simulink model "project"  (R2020a)
settings: Solver=VariableStepAuto  StartTime=0.0  StopTime=1000  RelTol=1e-3
values from neighbouring files (symbols this model uses):
  a = (6371+h)*1e3    (= 6871000)    [AMM_main.m]    (also in Data.m)
  A_RW = sqrt([prop1;prop2;prop3]/(prop1+prop2+prop3))    [AMM_main.m]    (also in Data.m)
  A_t = [Ax;Ay;Az;Ax;Ay;Az;A_sp;A_sp;A_sp;A_sp;]    [AMM_main.m]    (also in Data.m)
  alpha = 0.005    [AMM_main.m]    (also in Data.m = 0.5)
  cd = 2.2    [AMM_main.m]    (also in Data.m)
  horiz_ang_err = rand(3,1) - 0.5    [Data.m]
  horiz_err = 0.25*pi/180    (= 0.00436332312999)    [Data.m]
  init_DCM = DCM0_track    [AMM_main.m]    (also in Data.m = [0.097540404999410   0.957506835434298   0.970592781760616)
  init_orb = orb0_track    [AMM_main.m]    (also in Data.m = [e0,i0,O0,o0,th0])
  init_tumbl = w0_track    [AMM_main.m]    (also in Data.m = 10*pi/180*dir)
  Ir = 1e-7    (= 1e-07)    [AMM_main.m]    (also in Data.m)
  Iz = 2e-7    (= 2e-07)    [AMM_main.m]    (also in Data.m)
  J = [Jx;Jy;Jz]    [AMM_main.m]    (also in Data.m)
  K1 = .05    (= 0.05)    [AMM_main.m]    (also in Data.m)
  K2 = 0.5*K1^2    (= 0.00125)    [AMM_main.m]    (also in Data.m)
  magn_ang_err = rand(3,1) - 0.5    [Data.m]
  magn_err = 2*pi/180    (= 0.0349065850399)    [Data.m]
  max_mx = 1.19    [AMM_main.m]    (also in Data.m)
  max_my = 1.19    [AMM_main.m]    (also in Data.m)
  max_mz = 1.19    [AMM_main.m]    (also in Data.m)
  MS_freq = 1    [AMM_main.m]    (also in Data.m)
  mu = 3.986004418e14    (= 398600441800000)    [AMM_main.m]    (also in Data.m)
  n = sqrt( mu / a^3 )    [AMM_main.m]    (also in Data.m)
  rho = [rho_sMB;rho_dMB;rho_sSP;rho_dSP]    [AMM_main.m]    (also in Data.m)
  rho_air = 4.39e-16 * 1e6/1e3    (= 4.39e-13)    [AMM_main.m]    (also in Data.m)
  RW_Ir = 3.4e-4    (= 0.00034)    [AMM_main.m]    (also in Data.m)
  RW_max_momentum = 400e-3    (= 0.4)    [AMM_main.m]    (also in Data.m)
  RW_max_torque = 100e-3    (= 0.1)    [AMM_main.m]    (also in Data.m)
  wr = 100*pi/180    (= 1.74532925199)    [AMM_main.m]    (also in Data.m)
  ww_earth = 2*pi/(24*3600)*[0;0;1]    [AMM_main.m]    (also in Data.m)
libraries: vrlib x6, simulink x5, dspmtrx3 x2
(part 1 of 2)
settings Model: Creator=alejandrodemiguelmendiola  LastModifiedBy=alejandrodemiguelmendiola

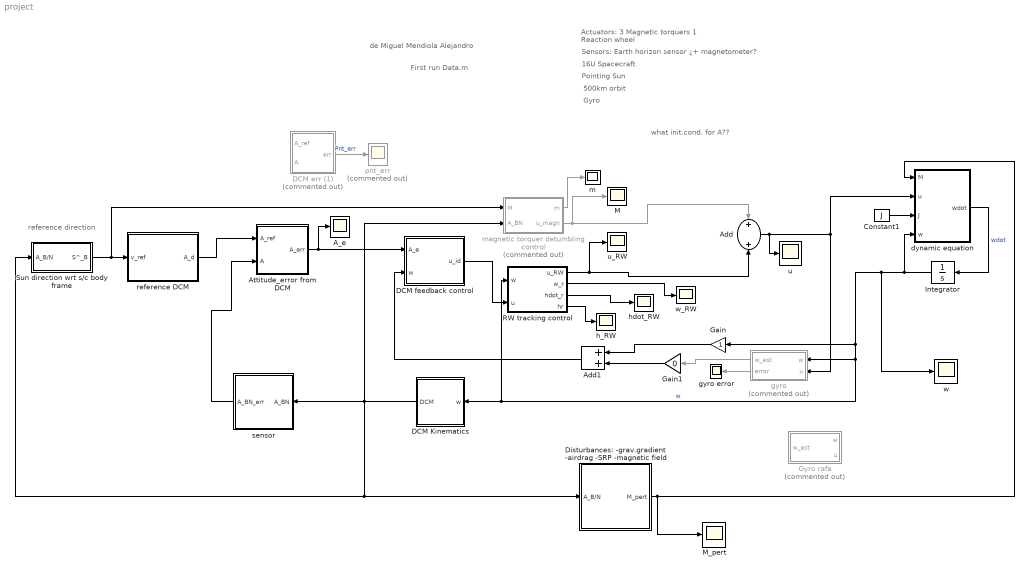
== system project ==
  note: reference direction
  note: what init.cond. for A??
  note: First run Data.m
  note: Gyro
  note: 500km orbit
  note: Pointing Sun
  note: 16U Spacecraft
  note: Sensors: Earth horizon sensor ¿+ magnetometer?
  note: Actuators: 3 Magnetic torquers
      | 		  1 Reaction wheel
  note: de Miguel Mendiola Alejandro
  A_e : Scope
  Add : Sum
  Add1 : Sum
  Attitude_error from DCM : Subsystem
  Constant1 : Constant  Value=J
  DCM Kinematics : Subsystem
  DCM err (1) : Subsystem  Commented=on
  DCM feedback control : Subsystem
  Disturbances: -grav.gradient -airdrag -SRP -magnetic field : Subsystem
  Gain : Gain
  Gain1 : Gain  Gain=0
  Gyro rafa : Subsystem  Commented=on
  Integrator : Integrator  InitialCondition=[1;1;1]*1e-3
  M : Scope
  M_pert : Scope
  RW tracking control : Subsystem
  Sun direction wrt s/c body frame : Subsystem
  dynamic equation : MATLAB Function  TreatAsAtomicUnit=on
  gyro : Subsystem  Commented=on
  gyro error : Scope
  h_RW : Scope
  hdot_RW : Scope
  m : Scope
  magnetic torquer detumbling control : Subsystem  Commented=on
  pnt_err : Scope  Commented=on
  reference DCM : Subsystem
  sensor : Subsystem
  u : Scope
  u_RW : Scope
  w : Scope
  w_RW : Scope
  wires:
  dynamic equation/1(wdot) -> Integrator/1  "wdot"
  Integrator/1 -> RW tracking control/1(w), DCM Kinematics/1(w), gyro/1(w), Gain/1, w/1, dynamic equation/4(w)  "w"
  Disturbances: -grav.gradient -airdrag -SRP -magnetic field/1(M_pert) -> dynamic equation/1(M), M_pert/1
  magnetic torquer detumbling control/2(u_magn) -> M/1, Add/1
  RW tracking control/1(u_RW) -> Add/2, u_RW/1
  Add/1 -> u/1, gyro/2(u), dynamic equation/2(u)
  gyro/2(error) -> gyro error/1
  RW tracking control/2(w_r) -> w_RW/1
  RW tracking control/3(hdot_r) -> hdot_RW/1
  Constant1/1 -> dynamic equation/3(J)
  RW tracking control/4(hr) -> h_RW/1
  Add1/1 -> DCM feedback control/2(w)
  Gain1/1 -> Add1/2
  gyro/1(w_est) -> Gain1/1
  Gain/1 -> Add1/1
  magnetic torquer detumbling control/1(m) -> m/1
  Sun direction wrt s/c body frame/1(S^_B) -> magnetic torquer detumbling control/1(M), reference DCM/1(v_ref)
  reference DCM/1(A_d) -> Attitude_error from DCM/1(A_ref)
  DCM feedback control/1(u_id) -> RW tracking control/2(u)
  DCM Kinematics/1(DCM) -> Sun direction wrt s/c body frame/1(A_B/N), Disturbances: -grav.gradient -airdrag -SRP -magnetic field/1(A_B/N), sensor/1(A_BN), magnetic torquer detumbling control/2(A_BN)
  Attitude_error from DCM/1(A_err) -> A_e/1, DCM feedback control/1(A_e)
  DCM err (1)/1(err) -> pnt_err/1  "Pnt_err"
  sensor/1(A_BN_err) -> Attitude_error from DCM/2(A)

== system project/Attitude_error from DCM ==
  A_ref : Inport
  A : Inport  Port=2
  Identity Matrix : dspmtrx3/Identity Matrix  Inherit=off  N=3  Ts=1  dataType=double  isSigned=on  wordLen=16  udDataType=sfix(16)  fracBitsMode=Best precision  numFracBits=15  OutDataTypeStr=double  LastOutDataTypeStr=double
  Matrix Multiply1 : Product  Multiplication=Matrix(*)
  Sum : Sum  Inputs=-+|
  Transpose1 : Math  Operator=transpose  SaturateOnIntegerOverflow=on
  A_err : Outport
  wires:
  Identity Matrix/1 -> Sum/1
  Matrix Multiply1/1 -> Sum/2
  A_ref/1 -> Transpose1/1
  Transpose1/1 -> Matrix Multiply1/2
  A/1 -> Matrix Multiply1/1
  Sum/1 -> A_err/1

== system project/DCM Kinematics ==
  w : Inport
  Integrator : Integrator  InitialCondition=init_DCM
  Iterative Orthonormalization : Subsystem
  Product1 : Product  Multiplication=Matrix(*)
  Unary Minus : UnaryMinus
  hat : MATLAB Function  TreatAsAtomicUnit=on
  DCM : Outport
  wires:
  Unary Minus/1 -> Integrator/1  "Adot"
  hat/1(w_hat) -> Product1/1
  Product1/1 -> Unary Minus/1
  w/1 -> hat/1(w)
  Iterative Orthonormalization/1(A_Ortho) -> Product1/2, DCM/1  "A_ortho"
  Integrator/1 -> Iterative Orthonormalization/1(A)  "A"

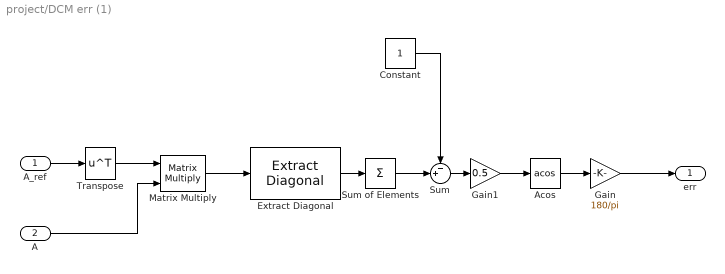
== system project/DCM err (1) ==
  A_ref : Inport
  A : Inport  Port=2
  Acos : Trigonometry  Operator=acos
  Constant : Constant
  Extract Diagonal : dspmtrx3/Extract Diagonal
      settings: SourceProductBaseCode=DS
  Gain : Gain  Gain=180/pi
  Gain1 : Gain  Gain=0.5
  Matrix Multiply : Product  Multiplication=Matrix(*)
  Sum : Sum  Inputs=-+|
  Sum of Elements : Sum  Inputs=+
  Transpose : Math  Operator=transpose  SaturateOnIntegerOverflow=on
  err : Outport
  wires:
  Transpose/1 -> Matrix Multiply/1
  Matrix Multiply/1 -> Extract Diagonal/1
  Extract Diagonal/1 -> Sum of Elements/1
  A/1 -> Matrix Multiply/2
  A_ref/1 -> Transpose/1
  Sum/1 -> Gain1/1
  Acos/1 -> Gain/1
  Sum of Elements/1 -> Sum/2
  Constant/1 -> Sum/1
  Gain/1 -> err/1
  Gain1/1 -> Acos/1

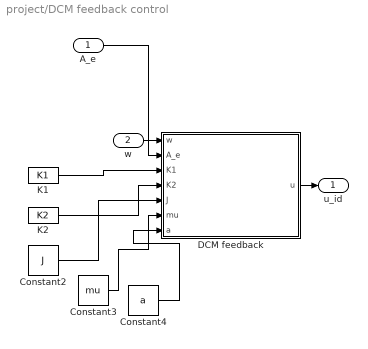
== system project/DCM feedback control ==
  A_e : Inport
  w : Inport  Port=2
  Constant2 : Constant  Value=J
  Constant3 : Constant  Value=mu
  Constant4 : Constant  Value=a
  DCM feedback : MATLAB Function  TreatAsAtomicUnit=on
  K1 : Constant  Value=K1
  K2 : Constant  Value=K2
  u_id : Outport
  wires:
  DCM feedback/1(u) -> u_id/1
  A_e/1 -> DCM feedback/2(A_e)
  Constant3/1 -> DCM feedback/6(mu)
  Constant2/1 -> DCM feedback/5(J)
  Constant4/1 -> DCM feedback/7(a)
  K2/1 -> DCM feedback/4(K2)
  w/1 -> DCM feedback/1(w)
  K1/1 -> DCM feedback/3(K1)

== system project/Disturbances: -grav.gradient -airdrag -SRP -magnetic field ==
  A_B/N : Inport
  Add : Sum  Inputs=++++
  SRP moment : Subsystem
  air drag : Subsystem
  gravity gradient : Subsystem
  magnetic torque : Subsystem
  M_pert : Outport
  wires:
  magnetic torque/1(magnetic torque M) -> Add/1
  SRP moment/1(T_srp) -> Add/2
  gravity gradient/1(G) -> Add/4
  Add/1 -> M_pert/1
  air drag/1(M_drag) -> Add/3
  A_B/N/1 -> magnetic torque/1(A_BN), SRP moment/1(A_B/N), gravity gradient/1(A_BN), air drag/1(A_B/N)

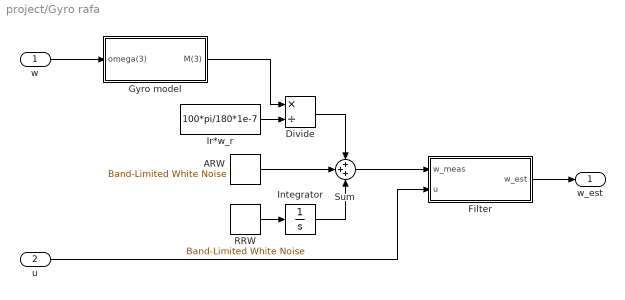
== system project/Gyro rafa ==
  w : Inport
  u : Inport  Port=2
  ARW : simulink/Sources/Band-Limited White Noise  Cov=1.9039e-09  Ts=0.0038168  seed=[23341]
  Divide : Product  Inputs=*/
  Filter : Subsystem
  Gyro model : Subsystem
  Integrator : Integrator  InitialCondition=pi/180/3600*[1 1 1]'
  Ir*w_r : Constant  Value=100*pi/180*1e-7
  RRW : simulink/Sources/Band-Limited White Noise  Cov=5.5423e-10  Ts=0.0038168  seed=[23341]
  Sum : Sum  Inputs=+++
  w_est : Outport
  wires:
  w/1 -> Gyro model/1(omega(3))
  Divide/1 -> Sum/1
  Sum/1 -> Filter/1(w_meas)
  Ir*w_r/1 -> Divide/2
  Gyro model/1(M(3)) -> Divide/1
  u/1 -> Filter/2(u)
  Filter/1(w_est) -> w_est/1
  ARW/1 -> Sum/2
  RRW/1 -> Integrator/1
  Integrator/1 -> Sum/3

== system project/RW tracking control ==
  w : Inport
  u : Inport  Port=2
  detumblingl control of 1 RW : Subsystem
  u_RW : Outport
  w_r : Outport  Port=2
  hdot_r : Outport  Port=3
  hr : Outport  Port=4
  wires:
  w/1 -> detumblingl control of 1 RW/1(w)
  detumblingl control of 1 RW/2(w_r) -> w_r/1
  detumblingl control of 1 RW/1(u_c) -> u_RW/1
  detumblingl control of 1 RW/4(hr) -> hr/1
  detumblingl control of 1 RW/3(hdot_r) -> hdot_r/1
  u/1 -> detumblingl control of 1 RW/2(u)

== system project/Sun direction wrt s//c body frame ==
  A_B/N : Inport
  Clock : Clock
  Product3 : Product  Multiplication=Matrix(*)
  Sun's direction : MATLAB Function  TreatAsAtomicUnit=on
  S^_B : Outport
  wires:
  Product3/1 -> S^_B/1
  A_B/N/1 -> Product3/1
  Clock/1 -> Sun's direction/1(t)
  Sun's direction/1(S_N) -> Product3/2  "S^_N"

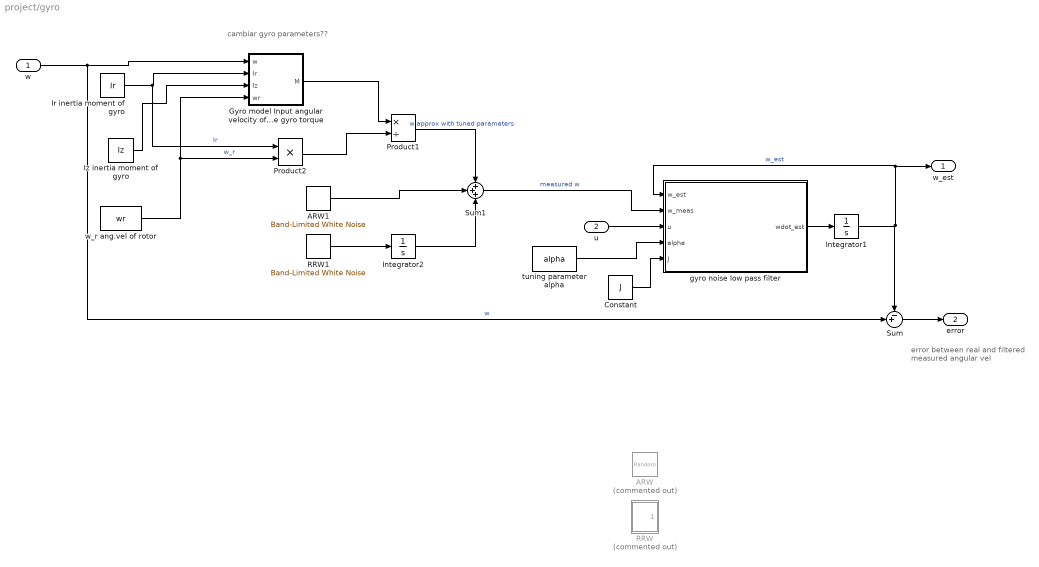
== system project/gyro ==
  note: cambiar gyro parameters??
  note: error between real
      | and filtered measured angular vel
  w : Inport
  u : Inport  Port=2
  ARW : RandomNumber  Commented=on  Variance=[1;1;1]*0.0025*pi/180  SampleTime=1/900  VectorParams1D=off
  ARW1 : simulink/Sources/Band-Limited White Noise  Cov=1.9039e-09  Ts=0.0038168  seed=[23341]
  Constant : Constant  Value=J
  Gyro model Input angular velocity of the spacecraft with output the gyro torque : Subsystem
  Integrator1 : Integrator  InitialCondition=init_tumbl
  Integrator2 : Integrator  InitialCondition=pi/180/3600*[1,1,1]'
  Ir inertia moment of gyro : Constant  Value=Ir
  Iz inertia moment of gyro : Constant  Value=Iz
  Product1 : Product  Inputs=*/
  Product2 : Product  Inputs=**
  RRW : Subsystem  Commented=on
  RRW1 : simulink/Sources/Band-Limited White Noise  Cov=5.5423e-10  Ts=0.0038168  seed=[23341]
  Sum : Sum  Inputs=-+|
  Sum1 : Sum  Inputs=+++
  gyro noise low pass filter : MATLAB Function  TreatAsAtomicUnit=on
  tuning parameter alpha : Constant  Value=alpha
  w_r ang.vel of rotor : Constant  Value=wr
  w_est : Outport
  error : Outport  Port=2
  wires:
  gyro noise low pass filter/1(wdot_est) -> Integrator1/1
  u/1 -> gyro noise low pass filter/3(u)
  tuning parameter alpha/1 -> gyro noise low pass filter/4(alpha)
  Sum/1 -> error/1
  Product2/1 -> Product1/2
  w/1 -> Gyro model Input angular velocity of the spacecraft with output the gyro torque/1(w), Sum/2  "w"
  Product1/1 -> Sum1/1  "w approx with tuned parameters"
  Integrator1/1 -> Sum/1, w_est/1, gyro noise low pass filter/1(w_est)  "w_est"
  Ir inertia moment of gyro/1 -> Product2/1, Gyro model Input angular velocity of the spacecraft with output the gyro torque/2(Ir)  "Ir"
  w_r ang.vel of rotor/1 -> Product2/2, Gyro model Input angular velocity of the spacecraft with output the gyro torque/4(wr)  "w_r"
  Iz inertia moment of gyro/1 -> Gyro model Input angular velocity of the spacecraft with output the gyro torque/3(Iz)
  Sum1/1 -> gyro noise low pass filter/2(w_meas)  "measured w"
  Gyro model Input angular velocity of the spacecraft with output the gyro torque/1(M) -> Product1/1
  Constant/1 -> gyro noise low pass filter/5(J)
  ARW1/1 -> Sum1/2
  RRW1/1 -> Integrator2/1
  Integrator2/1 -> Sum1/3

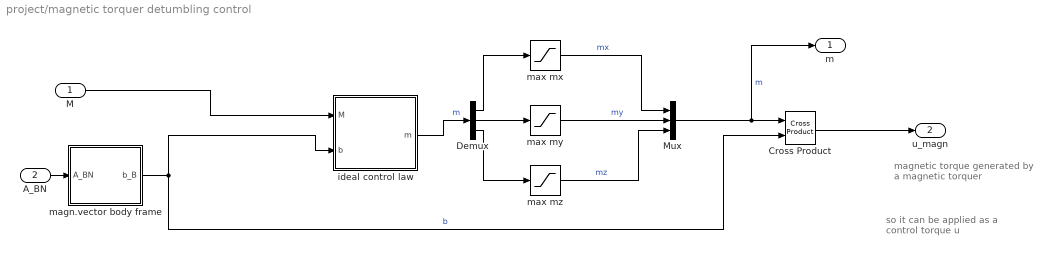
== system project/magnetic torquer detumbling control ==
  note: so it can be applied
      | as a control torque u
  note: magnetic torque
      | generated by a
      | magnetic torquer
  M : Inport
  A_BN : Inport  Port=2
  Cross Product : vrlib/Utilities/Cross Product
  Demux : Demux  Outputs=3
  Mux : Mux  Inputs=3
  ideal control law : MATLAB Function  TreatAsAtomicUnit=on
  magn.vector body frame : Subsystem
  max mx : Saturate  UpperLimit=max_mx  LowerLimit=-max_mx  ZeroCross=off
  max my : Saturate  UpperLimit=max_my  LowerLimit=-max_my  ZeroCross=off
  max mz : Saturate  UpperLimit=max_mz  LowerLimit=-max_mz  ZeroCross=off
  m : Outport
  u_magn : Outport  Port=2
  wires:
  ideal control law/1(m) -> Demux/1  "m"
  magn.vector body frame/1(b_B) -> ideal control law/2(b), Cross Product/2  "b"
  Mux/1 -> m/1, Cross Product/1  "m"
  Cross Product/1 -> u_magn/1
  max mx/1 -> Mux/1  "mx"
  max my/1 -> Mux/2  "my"
  max mz/1 -> Mux/3  "mz"
  Demux/1 -> max mx/1
  Demux/2 -> max my/1
  Demux/3 -> max mz/1
  M/1 -> ideal control law/1(M)
  A_BN/1 -> magn.vector body frame/1(A_BN)

== system project/reference DCM ==
  v_ref : Inport
  Constant2 : Constant  Value=a
  DCM_ref : MATLAB Function  TreatAsAtomicUnit=on
  Terminator : Terminator
  s/c position for a given orbit : Subsystem
  A_d : Outport
  wires:
  DCM_ref/1(A_BN) -> A_d/1
  Constant2/1 -> s/c position for a given orbit/1(a)
  v_ref/1 -> DCM_ref/1(v_ref)
  s/c position for a given orbit/1(r_N) -> DCM_ref/2(r_sc)
  s/c position for a given orbit/2(v_N) -> Terminator/1  "v_inertial"

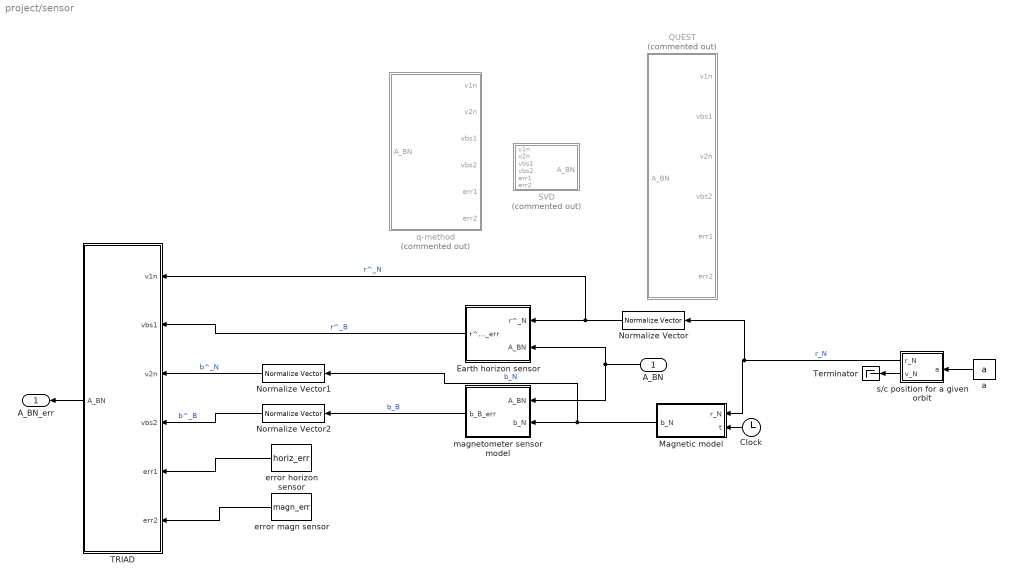
== system project/sensor ==
  A_BN : Inport
  Clock : Clock
  Earth horizon sensor : Subsystem
  Magnetic model : MATLAB Function  TreatAsAtomicUnit=on
  Normalize Vector : vrlib/Utilities/Normalize Vector  maxzero=0
  Normalize Vector1 : vrlib/Utilities/Normalize Vector  maxzero=0
  Normalize Vector2 : vrlib/Utilities/Normalize Vector  maxzero=0
  QUEST : MATLAB Function  Commented=on  TreatAsAtomicUnit=on
  SVD : MATLAB Function  Commented=on  TreatAsAtomicUnit=on
  TRIAD : MATLAB Function  TreatAsAtomicUnit=on
  Terminator : Terminator
  a : Constant  Value=a
  error horizon sensor : Constant  Value=horiz_err
  error magn sensor : Constant  Value=magn_err
  magnetometer sensor model : Subsystem
  q-method : MATLAB Function  Commented=on  TreatAsAtomicUnit=on
  s/c position for a given orbit : Subsystem
  A_BN_err : Outport
  wires:
  A_BN/1 -> Earth horizon sensor/2(A_BN), magnetometer sensor model/1(A_BN)
  Magnetic model/1(b_N) -> Normalize Vector1/1, magnetometer sensor model/2(b_N)  "b_N"
  Clock/1 -> Magnetic model/2(t)
  magnetometer sensor model/1(b_B_err) -> Normalize Vector2/1  "b_B"
  Earth horizon sensor/1(r^_B_err) -> TRIAD/2(vbs1)  "r^_B"
  TRIAD/1(A_BN) -> A_BN_err/1
  s/c position for a given orbit/2(v_N) -> Terminator/1
  a/1 -> s/c position for a given orbit/1(a)
  s/c position for a given orbit/1(r_N) -> Normalize Vector/1, Magnetic model/1(r_N)  "r_N"
  Normalize Vector/1 -> TRIAD/1(v1n), Earth horizon sensor/1(r^_N)  "r^_N"
  Normalize Vector2/1 -> TRIAD/4(vbs2)  "b^_B"
  Normalize Vector1/1 -> TRIAD/3(v2n)  "b^_N"
  error horizon sensor/1 -> TRIAD/5(err1)
  error magn sensor/1 -> TRIAD/6(err2)

== system project/DCM Kinematics/Iterative Orthonormalization ==
  note: Uncomment if needed
      | With 2 blocks working:
      | Error ~1e-16 up to t=1e6
      | Error ~1e-14 up to t=1e7
  A : Inport
  Ortho DCM : Subsystem
  Ortho DCM1 : Subsystem
  Ortho DCM2 : Subsystem  Commented=through
  Ortho DCM3 : Subsystem  Commented=through
  Ortho DCM4 : Subsystem  Commented=through
  A_Ortho : Outport
  wires:
  Ortho DCM1/1(A_ortho) -> Ortho DCM2/1(A)
  Ortho DCM/1(A_ortho) -> Ortho DCM1/1(A)
  Ortho DCM3/1(A_ortho) -> Ortho DCM4/1(A)
  Ortho DCM2/1(A_ortho) -> Ortho DCM3/1(A)
  A/1 -> Ortho DCM/1(A)
  Ortho DCM4/1(A_ortho) -> A_Ortho/1

== system project/Disturbances: -grav.gradient -airdrag -SRP -magnetic field/SRP moment ==
  A_B/N : Inport
  Area : Constant  Value=A_t
  SRP disturbance torque : MATLAB Function  TreatAsAtomicUnit=on
  Sun direction wrt s/c body frame : Subsystem
  optical properties : Constant  Value=rho
  T_srp : Outport
  wires:
  A_B/N/1 -> Sun direction wrt s/c body frame/1(A_B/N)
  SRP disturbance torque/1(T_srp) -> T_srp/1
  Sun direction wrt s/c body frame/1(S^_B) -> SRP disturbance torque/1(S_B)
  Area/1 -> SRP disturbance torque/2(A)
  optical properties/1 -> SRP disturbance torque/3(rho)

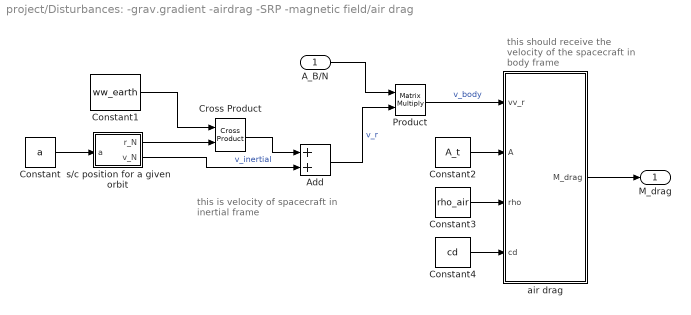
== system project/Disturbances: -grav.gradient -airdrag -SRP -magnetic field/air drag ==
  note: this is velocity
      | of spacecraft in
      | inertial frame
  note: this should receive the
      | velocity of the spacecraft
      | in body frame
  A_B/N : Inport
  Add : Sum
  Constant : Constant  Value=a
  Constant1 : Constant  Value=ww_earth
  Constant2 : Constant  Value=A_t
  Constant3 : Constant  Value=rho_air
  Constant4 : Constant  Value=cd
  Cross Product : vrlib/Utilities/Cross Product
  Product : Product  Multiplication=Matrix(*)
  air drag : MATLAB Function  TreatAsAtomicUnit=on
  s/c position for a given orbit : Subsystem
  M_drag : Outport
  wires:
  air drag/1(M_drag) -> M_drag/1
  A_B/N/1 -> Product/1
  Product/1 -> air drag/1(vv_r)  "v_body"
  Constant/1 -> s/c position for a given orbit/1(a)
  s/c position for a given orbit/1(r_N) -> Cross Product/2
  Constant1/1 -> Cross Product/1
  Cross Product/1 -> Add/1
  s/c position for a given orbit/2(v_N) -> Add/2  "v_inertial"
  Add/1 -> Product/2  "v_r"
  Constant2/1 -> air drag/2(A)
  Constant4/1 -> air drag/4(cd)
  Constant3/1 -> air drag/3(rho)

== system project/Disturbances: -grav.gradient -airdrag -SRP -magnetic field/gravity gradient ==
  A_BN : Inport
  A_N/L : Subsystem
  Product : Product  Multiplication=Matrix(*)
  gravity gradient : MATLAB Function  TreatAsAtomicUnit=on
  mean motion : Constant  Value=n
  moment of inertia : Constant  Value=J
  G : Outport
  wires:
  gravity gradient/1(G) -> G/1
  A_N/L/1(A_N/L) -> Product/2
  A_BN/1 -> Product/1
  Product/1 -> gravity gradient/1(A_BL)
  moment of inertia/1 -> gravity gradient/2(J)
  mean motion/1 -> gravity gradient/3(n)

== system project/Disturbances: -grav.gradient -airdrag -SRP -magnetic field/magnetic torque ==
  A_BN : Inport
  Cross Product : vrlib/Utilities/Cross Product
  m (worst case scenario) : Constant  Value=[0.1;0.1;0.1]
  m (from labs) : Constant  Commented=on  Value=[0.01;0.05;0.01]
  magnetic model : Subsystem
  magnetic torque M : Outport
  wires:
  magnetic model/1(b_B) -> Cross Product/2  "b_B"
  m (worst case scenario)/1 -> Cross Product/1
  Cross Product/1 -> magnetic torque M/1  "M"
  A_BN/1 -> magnetic model/1(A_BN)

== system project/Gyro rafa/Filter ==
  w_meas : Inport
  u : Inport  Port=2
  Integrator : Integrator  InitialCondition=[-0.0157; -0.1329; 0.1121]
  MATLAB Function : MATLAB Function  TreatAsAtomicUnit=on
  w_est : Outport
  wires:
  MATLAB Function/1(west_dot) -> Integrator/1
  Integrator/1 -> w_est/1, MATLAB Function/3(w_est)
  w_meas/1 -> MATLAB Function/1(w_meas)
  u/1 -> MATLAB Function/2(u)

== system project/Gyro rafa/Gyro model ==
  omega(3) : Inport
  Integrator : Integrator  InitialCondition=zeros(6,1)
  MATLAB Function : MATLAB Function  TreatAsAtomicUnit=on
  Scope : Scope
  Scope1 : Scope
  M(3) : Outport
  wires:
  MATLAB Function/2(M) -> M(3)/1
  omega(3)/1 -> MATLAB Function/2(w)
  MATLAB Function/1(x_dot) -> Scope/1, Integrator/1
  Integrator/1 -> Scope1/1, MATLAB Function/1(x)

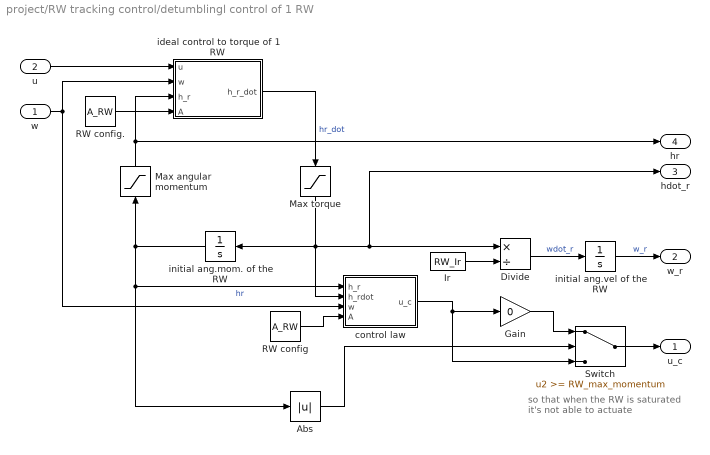
== system project/RW tracking control/detumblingl control of 1 RW ==
  note: so that when the RW is saturated
      | it's not able to actuate
  w : Inport
  u : Inport  Port=2
  Abs : Abs
  Divide : Product  Inputs=*/
  Gain : Gain  Gain=0
  Ir : Constant  Value=RW_Ir
  Max angular momentum : Saturate  UpperLimit=RW_max_momentum  LowerLimit=-RW_max_momentum
  Max torque : Saturate  UpperLimit=RW_max_torque  LowerLimit=-RW_max_torque  ZeroCross=off
  RW config : Constant  Value=A_RW
  RW config. : Constant  Value=A_RW
  Switch : Switch  Threshold=RW_max_momentum
  control law : MATLAB Function  TreatAsAtomicUnit=on
  ideal control to torque of 1 RW : MATLAB Function  TreatAsAtomicUnit=on
  "initial ang.mom. of the RW " : Integrator
  initial ang.vel of the RW : Integrator
  u_c : Outport
  w_r : Outport  Port=2
  hdot_r : Outport  Port=3
  hr : Outport  Port=4
  wires:
  u/1 -> ideal control to torque of 1 RW/1(u)
  w/1 -> ideal control to torque of 1 RW/2(w), control law/3(w)
  ideal control to torque of 1 RW/1(h_r_dot) -> Max torque/1  "hr_dot"
  "initial ang.mom. of the RW "/1 -> Max angular momentum/1, Abs/1, control law/1(h_r)  "hr"
  Max torque/1 -> "initial ang.mom. of the RW "/1, control law/2(h_rdot), hdot_r/1, Divide/1
  Max angular momentum/1 -> hr/1, ideal control to torque of 1 RW/3(h_r)
  Ir/1 -> Divide/2
  Divide/1 -> initial ang.vel of the RW/1  "wdot_r"
  initial ang.vel of the RW/1 -> w_r/1  "w_r"
  RW config/1 -> control law/4(A)
  RW config./1 -> ideal control to torque of 1 RW/4(A)
  Abs/1 -> Switch/2
  Switch/1 -> u_c/1
  control law/1(u_c) -> Gain/1, Switch/3
  Gain/1 -> Switch/1

== system project/gyro/Gyro model Input angular velocity of the spacecraft with output the gyro torque ==
  w : Inport
  Ir : Inport  Port=2
  Iz : Inport  Port=3
  wr : Inport  Port=4
  Integrator2 : Integrator  InitialCondition=[0;0;0;0;0;0]
  MATLAB Function1 : MATLAB Function  TreatAsAtomicUnit=on
  M : Outport
  wires:
  Integrator2/1 -> MATLAB Function1/4(x)
  MATLAB Function1/1(x_dot) -> Integrator2/1
  w/1 -> MATLAB Function1/5(w)
  MATLAB Function1/2(M) -> M/1
  Ir/1 -> MATLAB Function1/1(Ir)
  Iz/1 -> MATLAB Function1/2(Iz)
  wr/1 -> MATLAB Function1/3(w_r)

== system project/gyro/RRW ==
  Integrator2 : Integrator  InitialCondition=pi/180/3600*[1;1;1]
  Random Number : RandomNumber  Variance=1.5e-8*[1;1;1]  SampleTime=1/900  VectorParams1D=off
  RRW : Outport
  wires:
  Integrator2/1 -> RRW/1  "b"
  Random Number/1 -> Integrator2/1  "bdot"

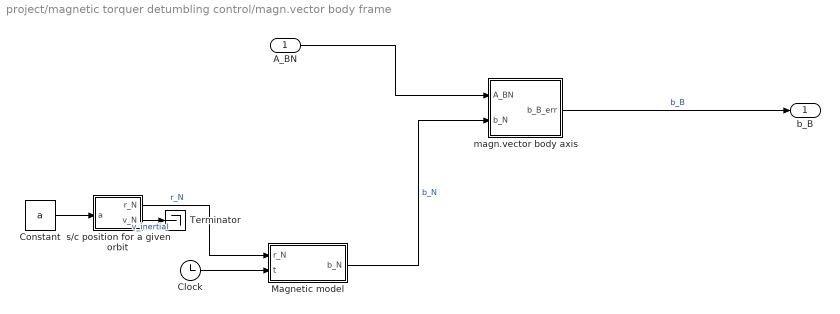
== system project/magnetic torquer detumbling control/magn.vector body frame ==
  A_BN : Inport
  Clock : Clock
  Constant : Constant  Value=a
  Magnetic model : MATLAB Function  TreatAsAtomicUnit=on
  Terminator : Terminator
  magn.vector body axis : Subsystem
  s/c position for a given orbit : Subsystem
  b_B : Outport
  wires:
  A_BN/1 -> magn.vector body axis/1(A_BN)
  magn.vector body axis/1(b_B_err) -> b_B/1  "b_B"
  Magnetic model/1(b_N) -> magn.vector body axis/2(b_N)  "b_N"
  s/c position for a given orbit/1(r_N) -> Magnetic model/1(r_N)  "r_N"
  Constant/1 -> s/c position for a given orbit/1(a)
  Clock/1 -> Magnetic model/2(t)
  s/c position for a given orbit/2(v_N) -> Terminator/1  "v_inertial"

== system project/reference DCM/s//c position for a given orbit ==
  a : Inport
  Earth's position : MATLAB Function  TreatAsAtomicUnit=on
  orb_elements dynamics : Subsystem
  r_N : Outport
  v_N : Outport  Port=2
  wires:
  Earth's position/1(r_N) -> r_N/1  "r_N"
  orb_elements dynamics/1(orb_elements) -> Earth's position/2(orb_elements)
  a/1 -> orb_elements dynamics/1(a), Earth's position/1(a)  "a"
  Earth's position/2(v_N) -> v_N/1

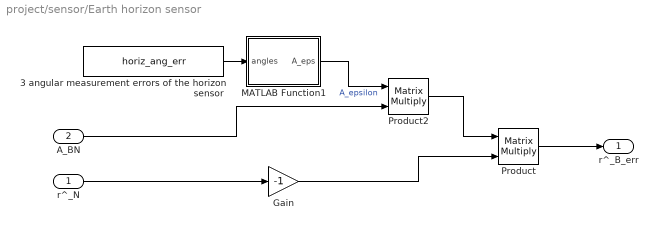
== system project/sensor/Earth horizon sensor ==
  r^_N : Inport
  A_BN : Inport  Port=2
  3 angular measurement errors of the horizon sensor : Constant  Value=horiz_ang_err
  Gain : Gain  Gain=-1
  MATLAB Function1 : MATLAB Function  TreatAsAtomicUnit=on
  Product : Product  Multiplication=Matrix(*)
  Product2 : Product  Multiplication=Matrix(*)
  r^_B_err : Outport
  wires:
  MATLAB Function1/1(A_eps) -> Product2/1  "A_epsilon"
  A_BN/1 -> Product2/2
  3 angular measurement errors of the horizon sensor/1 -> MATLAB Function1/1(angles)
  Product/1 -> r^_B_err/1
  Product2/1 -> Product/1
  r^_N/1 -> Gain/1
  Gain/1 -> Product/2

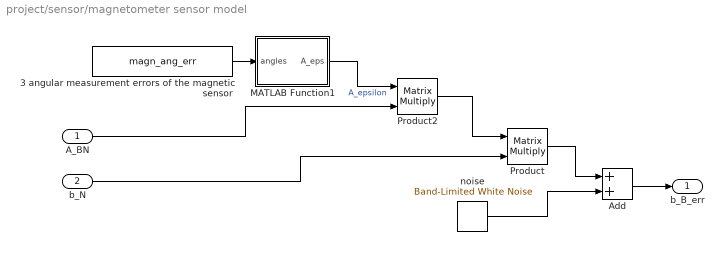
== system project/sensor/magnetometer sensor model ==
  A_BN : Inport
  b_N : Inport  Port=2
  3 angular measurement errors of the magnetic sensor : Constant  Value=magn_ang_err
  Add : Sum
  MATLAB Function1 : MATLAB Function  TreatAsAtomicUnit=on
  Product : Product  Multiplication=Matrix(*)
  Product2 : Product  Multiplication=Matrix(*)
  noise : simulink/Sources/Band-Limited White Noise  Cov=MS_noise  Ts=MS_freq  seed=[23341]
  b_B_err : Outport
  wires:
  MATLAB Function1/1(A_eps) -> Product2/1  "A_epsilon"
  A_BN/1 -> Product2/2
  3 angular measurement errors of the magnetic sensor/1 -> MATLAB Function1/1(angles)
  Product2/1 -> Product/1
  b_N/1 -> Product/2
  Add/1 -> b_B_err/1
  Product/1 -> Add/1
  noise/1 -> Add/2

== system project/sensor/s//c position for a given orbit ==
  a : Inport
  Earth's position : MATLAB Function  TreatAsAtomicUnit=on
  orb_elements dynamics : Subsystem
  r_N : Outport
  v_N : Outport  Port=2
  wires:
  Earth's position/1(r_N) -> r_N/1  "r_N"
  orb_elements dynamics/1(orb_elements) -> Earth's position/2(orb_elements)
  a/1 -> orb_elements dynamics/1(a), Earth's position/1(a)  "a"
  Earth's position/2(v_N) -> v_N/1

== system project/DCM Kinematics/Iterative Orthonormalization/Ortho DCM ==
  A : Inport
  Gain : Gain  Gain=1.5
  Gain1 : Gain  Gain=0.5
  Matrix Multiply : Product  Multiplication=Matrix(*)
  Matrix Multiply1 : Product  Multiplication=Matrix(*)
  Sum : Sum  Inputs=|+-
  Transpose : Math  Operator=transpose  SaturateOnIntegerOverflow=on
  A_ortho : Outport
  wires:
  Sum/1 -> A_ortho/1
  Gain/1 -> Sum/1
  A/1 -> Matrix Multiply1/2, Transpose/1, Matrix Multiply/1, Gain/1
  Gain1/1 -> Sum/2
  Transpose/1 -> Matrix Multiply/2
  Matrix Multiply/1 -> Matrix Multiply1/1
  Matrix Multiply1/1 -> Gain1/1

== system project/DCM Kinematics/Iterative Orthonormalization/Ortho DCM1 ==
  A : Inport
  Gain : Gain  Gain=1.5
  Gain1 : Gain  Gain=0.5
  Matrix Multiply : Product  Multiplication=Matrix(*)
  Matrix Multiply1 : Product  Multiplication=Matrix(*)
  Sum : Sum  Inputs=|+-
  Transpose : Math  Operator=transpose  SaturateOnIntegerOverflow=on
  A_ortho : Outport
  wires:
  Sum/1 -> A_ortho/1
  Gain/1 -> Sum/1
  A/1 -> Matrix Multiply1/2, Transpose/1, Matrix Multiply/1, Gain/1
  Gain1/1 -> Sum/2
  Transpose/1 -> Matrix Multiply/2
  Matrix Multiply/1 -> Matrix Multiply1/1
  Matrix Multiply1/1 -> Gain1/1

== system project/DCM Kinematics/Iterative Orthonormalization/Ortho DCM2 ==
  A : Inport
  Gain : Gain  Gain=1.5
  Gain1 : Gain  Gain=0.5
  Matrix Multiply : Product  Multiplication=Matrix(*)
  Matrix Multiply1 : Product  Multiplication=Matrix(*)
  Sum : Sum  Inputs=|+-
  Transpose : Math  Operator=transpose  SaturateOnIntegerOverflow=on
  A_ortho : Outport
  wires:
  Sum/1 -> A_ortho/1
  Gain/1 -> Sum/1
  A/1 -> Matrix Multiply1/2, Transpose/1, Matrix Multiply/1, Gain/1
  Gain1/1 -> Sum/2
  Transpose/1 -> Matrix Multiply/2
  Matrix Multiply/1 -> Matrix Multiply1/1
  Matrix Multiply1/1 -> Gain1/1

== system project/DCM Kinematics/Iterative Orthonormalization/Ortho DCM3 ==
  A : Inport
  Gain : Gain  Gain=1.5
  Gain1 : Gain  Gain=0.5
  Matrix Multiply : Product  Multiplication=Matrix(*)
  Matrix Multiply1 : Product  Multiplication=Matrix(*)
  Sum : Sum  Inputs=|+-
  Transpose : Math  Operator=transpose  SaturateOnIntegerOverflow=on
  A_ortho : Outport
  wires:
  Sum/1 -> A_ortho/1
  Gain/1 -> Sum/1
  A/1 -> Matrix Multiply1/2, Transpose/1, Matrix Multiply/1, Gain/1
  Gain1/1 -> Sum/2
  Transpose/1 -> Matrix Multiply/2
  Matrix Multiply/1 -> Matrix Multiply1/1
  Matrix Multiply1/1 -> Gain1/1

== system project/DCM Kinematics/Iterative Orthonormalization/Ortho DCM4 ==
  A : Inport
  Gain : Gain  Gain=1.5
  Gain1 : Gain  Gain=0.5
  Matrix Multiply : Product  Multiplication=Matrix(*)
  Matrix Multiply1 : Product  Multiplication=Matrix(*)
  Sum : Sum  Inputs=|+-
  Transpose : Math  Operator=transpose  SaturateOnIntegerOverflow=on
  A_ortho : Outport
  wires:
  Sum/1 -> A_ortho/1
  Gain/1 -> Sum/1
  A/1 -> Matrix Multiply1/2, Transpose/1, Matrix Multiply/1, Gain/1
  Gain1/1 -> Sum/2
  Transpose/1 -> Matrix Multiply/2
  Matrix Multiply/1 -> Matrix Multiply1/1
  Matrix Multiply1/1 -> Gain1/1

== system project/Disturbances: -grav.gradient -airdrag -SRP -magnetic field/SRP moment/Sun direction wrt s//c body frame ==
  A_B/N : Inport
  Clock : Clock
  Product3 : Product  Multiplication=Matrix(*)
  Sun's direction : MATLAB Function  TreatAsAtomicUnit=on
  S^_B : Outport
  wires:
  Product3/1 -> S^_B/1
  A_B/N/1 -> Product3/1
  Clock/1 -> Sun's direction/1(t)
  Sun's direction/1(S_N) -> Product3/2  "S^_N"

== system project/Disturbances: -grav.gradient -airdrag -SRP -magnetic field/air drag/s//c position for a given orbit ==
  a : Inport
  Earth's position : MATLAB Function  TreatAsAtomicUnit=on
  orb_elements dynamics : Subsystem
  r_N : Outport
  v_N : Outport  Port=2
  wires:
  Earth's position/1(r_N) -> r_N/1  "r_N"
  orb_elements dynamics/1(orb_elements) -> Earth's position/2(orb_elements)
  a/1 -> orb_elements dynamics/1(a), Earth's position/1(a)  "a"
  Earth's position/2(v_N) -> v_N/1

== system project/Disturbances: -grav.gradient -airdrag -SRP -magnetic field/gravity gradient/A_N//L ==
  Clock : Clock
  MATLAB Function1 : MATLAB Function  TreatAsAtomicUnit=on
  Transpose : Math  Operator=transpose  SaturateOnIntegerOverflow=on
  mean motion : Constant  Value=n
  A_N/L : Outport
  wires:
  Transpose/1 -> A_N/L/1  "A_N/L"
  Clock/1 -> MATLAB Function1/1(t)
  MATLAB Function1/1(A_LN) -> Transpose/1  "A_LN"
  mean motion/1 -> MATLAB Function1/2(n)

== system project/Disturbances: -grav.gradient -airdrag -SRP -magnetic field/magnetic torque/magnetic model ==
  A_BN : Inport
  Clock : Clock
  Constant : Constant  Value=a
  Magnetic model : MATLAB Function  TreatAsAtomicUnit=on
  Terminator : Terminator
  magnetometer sensor model : Subsystem
  s/c position for a given orbit : Subsystem
  b_B : Outport
  wires:
  magnetometer sensor model/1(b_B) -> b_B/1  "b_B"
  Magnetic model/1(b_N) -> magnetometer sensor model/2(b_N)  "b_N"
  A_BN/1 -> magnetometer sensor model/1(A_BN)
  s/c position for a given orbit/1(r_N) -> Magnetic model/1(r_N)
  Clock/1 -> Magnetic model/2(t)
  Constant/1 -> s/c position for a given orbit/1(a)
  s/c position for a given orbit/2(v_N) -> Terminator/1  "v_inertial"

== system project/magnetic torquer detumbling control/magn.vector body frame/magn.vector body axis ==
  A_BN : Inport
  b_N : Inport  Port=2
  Product : Product  Multiplication=Matrix(*)
  b_B_err : Outport
  wires:
  A_BN/1 -> Product/1
  b_N/1 -> Product/2
  Product/1 -> b_B_err/1

== system project/magnetic torquer detumbling control/magn.vector body frame/s//c position for a given orbit ==
  a : Inport
  Earth's position : MATLAB Function  TreatAsAtomicUnit=on
  orb_elements dynamics : Subsystem
  r_N : Outport
  v_N : Outport  Port=2
  wires:
  Earth's position/1(r_N) -> r_N/1  "r_N"
  orb_elements dynamics/1(orb_elements) -> Earth's position/2(orb_elements)
  a/1 -> orb_elements dynamics/1(a), Earth's position/1(a)  "a"
  Earth's position/2(v_N) -> v_N/1

== system project/reference DCM/s//c position for a given orbit/orb_elements dynamics ==
  a : Inport
  Integrator : Integrator  InitialCondition=init_orb
  sat motion : MATLAB Function  TreatAsAtomicUnit=on
  orb_elements : Outport
  wires:
  Integrator/1 -> sat motion/2(orb_elements), orb_elements/1  "orb_elements"
  sat motion/1(orb_elements_dot) -> Integrator/1
  a/1 -> sat motion/1(a)

== system project/sensor/s//c position for a given orbit/orb_elements dynamics ==
  a : Inport
  Integrator : Integrator  InitialCondition=init_orb
  sat motion : MATLAB Function  TreatAsAtomicUnit=on
  orb_elements : Outport
  wires:
  Integrator/1 -> sat motion/2(orb_elements), orb_elements/1  "orb_elements"
  sat motion/1(orb_elements_dot) -> Integrator/1
  a/1 -> sat motion/1(a)

== system project/Disturbances: -grav.gradient -airdrag -SRP -magnetic field/air drag/s//c position for a given orbit/orb_elements dynamics ==
  a : Inport
  Integrator : Integrator  InitialCondition=init_orb
  sat motion : MATLAB Function  TreatAsAtomicUnit=on
  orb_elements : Outport
  wires:
  Integrator/1 -> sat motion/2(orb_elements), orb_elements/1  "orb_elements"
  sat motion/1(orb_elements_dot) -> Integrator/1
  a/1 -> sat motion/1(a)

== system project/Disturbances: -grav.gradient -airdrag -SRP -magnetic field/magnetic torque/magnetic model/magnetometer sensor model ==
  A_BN : Inport
  b_N : Inport  Port=2
  Product : Product  Multiplication=Matrix(*)
  b_B : Outport
  wires:
  A_BN/1 -> Product/1
  b_N/1 -> Product/2
  Product/1 -> b_B/1

== system project/Disturbances: -grav.gradient -airdrag -SRP -magnetic field/magnetic torque/magnetic model/s//c position for a given orbit ==
  a : Inport
  Earth's position : MATLAB Function  TreatAsAtomicUnit=on
  orb_elements dynamics : Subsystem
  r_N : Outport
  v_N : Outport  Port=2
  wires:
  Earth's position/1(r_N) -> r_N/1  "r_N"
  orb_elements dynamics/1(orb_elements) -> Earth's position/2(orb_elements)
  a/1 -> orb_elements dynamics/1(a), Earth's position/1(a)  "a"
  Earth's position/2(v_N) -> v_N/1

== system project/magnetic torquer detumbling control/magn.vector body frame/s//c position for a given orbit/orb_elements dynamics ==
  a : Inport
  Integrator : Integrator  InitialCondition=init_orb
  sat motion : MATLAB Function  TreatAsAtomicUnit=on
  orb_elements : Outport
  wires:
  Integrator/1 -> sat motion/2(orb_elements), orb_elements/1  "orb_elements"
  sat motion/1(orb_elements_dot) -> Integrator/1
  a/1 -> sat motion/1(a)

== system project/Disturbances: -grav.gradient -airdrag -SRP -magnetic field/magnetic torque/magnetic model/s//c position for a given orbit/orb_elements dynamics ==
  a : Inport
  Integrator : Integrator  InitialCondition=init_orb
  sat motion : MATLAB Function  TreatAsAtomicUnit=on
  orb_elements : Outport
  wires:
  Integrator/1 -> sat motion/2(orb_elements), orb_elements/1  "orb_elements"
  sat motion/1(orb_elements_dot) -> Integrator/1
  a/1 -> sat motion/1(a)

== matlab function project/gyro/Gyro model Input angular velocity of the spacecraft with output the gyro torque/MATLAB Function1 ==
  data: Ir input; Iz input; w_r input; x input; w input; x_dot output; M output
function [x_dot,M]  = Gyro(Ir,Iz,w_r,x,w)
%DATA
% Ir = 1e-7; %gyro inertia parameters 
% Iz = 2e-7;
% w_r = 100*pi/180; %angular velocity of gyro wheel
k_gyro=10; %tuning parameter for visco-elastic reaction torque
c_gyro = 2*sqrt(k_gyro*Iz); 


%tuning law for c for fastest convergence
w_x = w(1); %angular velocity in body frame 
w_y = w(2); 
w_z = w(3); 

% defining the theta_i and \dot theta_i 
x_dot = zeros(6,1); % x will be the state variable
th_x = x(1); %turning angle of the gyro
th_y = x(2); 
th_z = x(3);
va_x = x(4); %angular velocity of the gyro
va_y = x(5); 
va_z = x(6); 

%3 gyro dynamics expressed as 1st order differential equation
x_dot(1) = va_x;
x_dot(2) = va_y; 
x_dot(3) = va_z;
x_dot(4) = -(c_gyro/Iz)*va_x-(k_gyro/Iz)*th_x-(Ir/Iz)*w_r*w_x;
x_dot(5) = -(c_gyro/Iz)*va_y-(k_gyro/Iz)*th_y-(Ir/Iz)*w_r*w_y;
x_dot(6) = -(c_gyro/Iz)*va_z-(k_gyro/Iz)*th_z-(Ir/Iz)*w_r*w_z;


%feedback torque applied to the gyros 
M = zeros(3,1);
M(1) = -k_gyro*th_x-c_gyro*va_x;
M(2) = -k_gyro*th_y-c_gyro*va_y;
M(3) = -k_gyro*th_z-c_gyro*va_z;


end %function

== matlab function project/gyro/gyro noise low pass filter ==
  data: w_est input; w_meas input; u input; wdot_est output; alpha input; J input
function wdot_est = fcn(w_est,w_meas,u,alpha,J)

% J1 = 100.9e-2;
% J2 =  25.1e-2;
% J3 =  91.6e-2;
J1 = J(1);
J2 = J(2);
J3 = J(3);

wdot_est = zeros(size(w_est));

wdot_est(1) =       (J2 - J3)/J1 * w_est(2) * w_est(3) + u(1)/J1 - ...
                alpha*(w_est(1)-w_meas(1))/J1;
wdot_est(2) =       (J3 - J1)/J2 * w_est(1) * w_est(3) + u(2)/J2 - ...
                alpha*(w_est(2)-w_meas(2))/J2;
wdot_est(3) =       (J1 - J2)/J3 * w_est(1) * w_est(2) + u(3)/J3 - ...
                alpha*(w_est(3)-w_meas(3))/J3;

    
end

== matlab function project/sensor/magnetometer sensor model/MATLAB Function1 ==
  data: angles input; A_eps output
function A_eps = sens_err(angles)

phi   = angles(1);
theta = angles(2);
xi    = angles(3);


A_eps      = eye(3);

A_eps(1,1) =   cos(xi)*cos(theta);
A_eps(1,2) =   cos(xi)*sin(theta)*sin(phi) + sin(xi)*cos(phi);
A_eps(1,3) = - cos(xi)*sin(theta)*cos(phi) + sin(xi)*sin(phi);
A_eps(2,1) = - sin(xi)*cos(theta);
A_eps(2,2) = - sin(xi)*sin(theta)*sin(phi) + cos(xi)*cos(phi);
A_eps(2,3) =   sin(xi)*sin(theta)*cos(phi) + cos(xi)*sin(phi);
A_eps(3,1) =   sin(theta);
A_eps(3,2) = - cos(theta)*sin(phi);
A_eps(3,3) =   cos(theta)*cos(phi);

== matlab function project/sensor/Earth horizon sensor/MATLAB Function1 ==
  data: angles input; A_eps output
function A_eps = sens_err(angles)

phi   = angles(1);
theta = angles (2);
xi    = angles(3);


A_eps      = eye(3);

A_eps(1,1) =   cos(xi)*cos(theta);
A_eps(1,2) =   cos(xi)*sin(theta)*sin(phi) + sin(xi)*cos(phi);
A_eps(1,3) = - cos(xi)*sin(theta)*cos(phi) + sin(xi)*sin(phi);
A_eps(2,1) = - sin(xi)*cos(theta);
A_eps(2,2) = - sin(xi)*sin(theta)*sin(phi) + cos(xi)*cos(phi);
A_eps(2,3) =   sin(xi)*sin(theta)*cos(phi) + cos(xi)*sin(phi);
A_eps(3,1) =   sin(theta);
A_eps(3,2) = - cos(theta)*sin(phi);
A_eps(3,3) =   cos(theta)*cos(phi);

== matlab function project/RW tracking control/detumblingl control of 1 RW/control law ==
  data: h_r input; h_rdot input; w input; u_c output; A input
function u_c = fcn(h_r,h_rdot,w,A)

u_c = zeros(3,1);
u_c = -A*h_rdot-cross(w,A*h_r);

== matlab function project/sensor/Magnetic model ==
  data: r_N input; b_N output; t input
function b_N = fcn(r_N,t)
% coefficients
IGRF = '2000';
switch IGRF
    case '1995'
        g0_1 = -29682e-9;
        g1_1 = -1789e-9;
        h1_1 = 5318e-9;
    case '2000'
        g0_1 = -29615e-9;
        g1_1 = -1728e-9;
        h1_1 = 5186e-9;
end


w = 360/(24*3600) * pi/180; %[rad/s] angular rotation speed of Earth
decl = 11.5*pi/180; %[rad]
R = 6371.2e3; %equatorial radius [m]
r = norm(r_N);
rr_unit = r_N/r; %unitary vector

H0 = sqrt(g0_1^2 + g1_1^2 + h1_1^2);
m = [
    sin(decl)*cos(w*t);
    sin(decl)*sin(w*t);
    cos(decl)
    ]; %unit vector along dipole axis

b_N = R^3*H0/r^3*(3*(dot(m,rr_unit))*rr_unit - m); %Earth's MF in the inertial frame

== matlab function project/sensor/q-method ==
  data: v1n input; A_BN output; v2n input; vbs1 input; vbs2 input; err1 input; err2 input
function A_BN = fcn(v1n,v2n,vbs1,vbs2,err1,err2) %vb is not needed


% Attitude determination with q-method

% %% Data
% % From on-board models (inertial frame)
% v1n  = [ 0.2673; 0.5345; 0.8018];
% v2n  = [-0.3124; 0.9370; 0.1562];
% % From body-fixed sensors
%     % Perfect readings
% v1b  = [ 0.7749; 0.3447; 0.5297];
% v2b  = [ 0.6295; 0.6944;-0.3486];
%     % Actual readings (with errors)
% vbs1 = [ 0.7835; 0.3690; 0.4971];
% % vbs1  = [ 0.7749; 0.3447; 0.5297];
% err1 = 5; % degs
% vbs2 = [ 0.6272; 0.6965;-0.3484];
% % vbs2  = [ 0.6295; 0.6944;-0.3486];
% err2 = 1/8; % degs

%% q-method

alpha = [1/err1; 1/err2];
alpha = alpha/norm(alpha);

B = alpha(1)*vbs1*v1n' + alpha(2)*vbs2*v2n';
S = B + B';
Z = [ B(2,3)-B(3,2); B(3,1)-B(1,3); B(1,2)-B(2,1) ];
sigma = trace(B);

K = zeros(4);
K(1:3,1:3) = S-sigma*eye(3);
K(1:3, 4 ) = Z;
K( 4 ,1:3) = Z';
K( 4 , 4 ) = sigma;

[Evec, Eval] = eig(K);

q = Evec(:,4);

A_BN = zeros(3);

A_BN(1,1) = q(1)^2 - q(2)^2 - q(3)^2 + q(4)^2;
A_BN(1,2) = 2 * ( q(1)*q(2) + q(3)*q(4) );
A_BN(1,3) = 2 * ( q(1)*q(3) - q(2)*q(4) );
A_BN(2,1) = 2 * ( q(1)*q(2) - q(3)*q(4) );
A_BN(2,2) = - q(1)^2 + q(2)^2 - q(3)^2 + q(4)^2;
A_BN(2,3) = 2 * ( q(2)*q(3) + q(1)*q(4) );
A_BN(3,1) = 2 * ( q(1)*q(3) + q(2)*q(4) );
A_BN(3,2) = 2 * ( q(2)*q(3) - q(1)*q(4) );
A_BN(3,3) = - q(1)^2 - q(2)^2 + q(3)^2 + q(4)^2;
end

== matlab function project/Disturbances: -grav.gradient -airdrag -SRP -magnetic field/SRP moment/Sun direction wrt s//c body frame/Sun's direction ==
  data: t input; S_N output
function S_N = fcn(t)

%% data
Rs = 149597870700; %[m] but we can substitute it by 1 so we have a unitary vector
Rs = 1;
epsilon = 23.45 * pi/180; %[rad]
T = 365.25*24*3600; %[s]
nsun = 2*pi/T; % [s^-1]

%% 
S_N = Rs * [cos(nsun*t);
            sin(nsun*t)*cos(epsilon);
            sin(nsun*t)*sin(epsilon);];

end

== matlab function project/sensor/SVD ==
  data: v1n input; A_BN output; v2n input; vbs1 input; vbs2 input; err1 input; err2 input
function A_BN = fcn(v1n,v2n,vbs1,vbs2,err1,err2) %vb is not needed

% Attitude determination with SVD method

% %% Data
% % From on-board models (inertial frame)
% v1n  = [ 0.2673; 0.5345; 0.8018];
% v2n  = [-0.3124; 0.9370; 0.1562];
% % From body-fixed sensors
%     % Perfect readings
% v1b  = [ 0.7749; 0.3447; 0.5297];
% v2b  = [ 0.6295; 0.6944;-0.3486];
%     % Actual readings (with errors)
% vbs1 = [ 0.7835; 0.3690; 0.4971];
% % vbs1  = [ 0.7749; 0.3447; 0.5297];
% err1 = 5; % degs
% vbs2 = [ 0.6272; 0.6965;-0.3484];
% % vbs2  = [ 0.6295; 0.6944;-0.3486];
% err2 = 1/8; % degs

%% Single Value Decomposition method

alpha = [1/err1; 1/err2];
alpha = alpha/norm(alpha);

B = alpha(1)*vbs1*v1n' + alpha(2)*vbs2*v2n';

[U, S, V] = svd(B);
M = diag([1, 1, det(U)*det(V)]);

A_BN = U*M*V';

end

== matlab function project/sensor/QUEST ==
  data: v1n input; vbs1 input; A_BN output; v2n input; vbs2 input; err1 input; err2 input
function A_BN = fcn(v1n,vbs1,v2n,vbs2,err1,err2) %%vb is not needed

% Attitude determination with QUEST-method

% %% Data
% % From on-board models (inertial frame)
% v1n  = [ 0.2673; 0.5345; 0.8018];
% v2n  = [-0.3124; 0.9370; 0.1562];
% % From body-fixed sensors
%     % Perfect readings
% v1b  = [ 0.7749; 0.3447; 0.5297];
% v2b  = [ 0.6295; 0.6944;-0.3486];
%     % Actual readings (with errors)
% vbs1 = [ 0.7835; 0.3690; 0.4971];
% % vbs1  = [ 0.7749; 0.3447; 0.5297];
% err1 = 5; % degs
% vbs2 = [ 0.6272; 0.6965;-0.3484];
% % vbs2  = [ 0.6295; 0.6944;-0.3486];
% err2 = 1/8; % degs

%% QUEST method

alpha = [1/err1; 1/err2];
alpha = alpha/sum(alpha);

B = alpha(1)*vbs1*v1n' + alpha(2)*vbs2*v2n';
S = B + B';
Z = [ B(2,3)-B(3,2); B(3,1)-B(1,3); B(1,2)-B(2,1) ];
sigma = trace(B);

g = linsolve ( S - (sigma+1)*eye(3), - Z);

A_BN = zeros(3);

A_BN(1,1) = g(1)^2 - g(2)^2 - g(3)^2 + 1;
A_BN(1,2) = 2 * ( g(1)*g(2) + g(3) );
A_BN(1,3) = 2 * ( g(1)*g(3) - g(2) );
A_BN(2,1) = 2 * ( g(1)*g(2) - g(3) );
A_BN(2,2) = - g(1)^2 + g(2)^2 - g(3)^2 + 1;
A_BN(2,3) = 2 * ( g(2)*g(3) + g(1) );
A_BN(3,1) = 2 * ( g(1)*g(3) + g(2) );
A_BN(3,2) = 2 * ( g(2)*g(3) - g(1) );
A_BN(3,3) = - g(1)^2 - g(2)^2 + g(3)^2 + 1;

A_BN = A_BN / ( g(1)^2 + g(2)^2 + g(3)^2 + 1); %is this to normalize?

end

== matlab function project/sensor/TRIAD ==
  data: v1n input; vbs1 input; v2n input; vbs2 input; A_BN output; err1 input; err2 input
function A_BN = TRIAD(v1n,vbs1,v2n,vbs2,err1,err2)

if err1 < err2 %to ensure that the 1st measurement is lower error
    s1 = vbs1/norm(vbs1); % 1st is taken the measurement with lower error
    s2 = cross(vbs1,vbs2)/norm(cross(vbs1,vbs2));
    s3 = cross(s1,s2);

    v1 = v1n/norm(v1n);
    v2 = cross(v1n,v2n)/norm(cross(v1n,v2n));
    v3 = cross(v1,v2);
else
    s1 = vbs2/norm(vbs2); % 1st is taken the measurement with lower error
    s2 = cross(vbs2,vbs1)/norm(cross(vbs2,vbs1));
    s3 = cross(s1,s2);

    v1 = v2n/norm(v2n);
    v2 = cross(v2n,v1n)/norm(cross(v2n,v1n));
    v3 = cross(v1,v2);
end

A_BN = [s1, s2, s3] * [v1, v2, v3]';

end

== matlab function project/sensor/s//c position for a given orbit/Earth's position ==
  data: a input; orb_elements input; r_N output; v_N output
function [r_N,v_N]  = Earth_pos(a,orb_elements)

mu = 3.986004418e14;

e_mod = orb_elements(1);
i     = orb_elements(2);
Omega = orb_elements(3);
omega = orb_elements(4);
theta = orb_elements(5);


h_mod = sqrt(mu*a*(1-e_mod^2));
    
e_unit = rotation_matrix_R3(-Omega) * ...
         rotation_matrix_R1(-i) * ...
         rotation_matrix_R3(-omega) * [1;0;0];
p_unit = rotation_matrix_R3(-Omega) * ...
         rotation_matrix_R1(-i) * ...
         rotation_matrix_R3(-omega) * [0;1;0];
     
r_mod_0 = h_mod^2/mu/(1+e_mod*cos(theta));
r_N       = r_mod_0 * ( cos(theta) * e_unit  +  sin(theta) * p_unit );
v_r     = mu/h_mod * e_mod*sin(theta);
v_theta = mu/h_mod * (1 + e_mod*cos(theta));
v_N       = v_r     * (  cos(theta) * e_unit  +  sin(theta) * p_unit )+ ...
          v_theta * ( -sin(theta) * e_unit  +  cos(theta) * p_unit );
end


function R1 = rotation_matrix_R1(alpha)
%{
rotation_matrix_R1: computes rotation matrix of angle alpha around x axis

INPUT:
	alpha[1]                Angle rotated
                                [rad]

OUTPUT:
    R1 [3x3]                Rotation matrix
                                [(3x3) x -]
%}

R1 = zeros(3);

R1(1,1) = 1;
R1(2,2) =  cos(alpha);
R1(2,3) =  sin(alpha);
R1(3,2) = -sin(alpha);
R1(3,3) =  cos(alpha);
end


function R3 = rotation_matrix_R3(alpha)
%{
rotation_matrix_R3: computes rotation matrix of angle alpha around z axis

INPUT:
	alpha[1]                Angle rotated
                                [rad]

OUTPUT:
    R3 [3x3]                Rotation matrix
                                [(3x3) x -]

%}

R3 = zeros(3);

R3(1,1) =  cos(alpha);
R3(1,2) =  sin(alpha);
R3(2,1) = -sin(alpha);
R3(2,2) =  cos(alpha);
R3(3,3) =  1;
end

== matlab function project/sensor/s//c position for a given orbit/orb_elements dynamics/sat motion ==
  data: a input; orb_elements input; orb_elements_dot output
function orb_elements_dot = orbit(a,orb_elements)

mu = 3.986004418e14;

e     = orb_elements(1);
i     = orb_elements(2);
O = orb_elements(3);
o = orb_elements(4);
theta = orb_elements(5); %true anomaly


n     = sqrt( mu / a^3 ); %mean motion: angular speed required to complete 1 orbit

orb_elements_dot    = zeros (size(orb_elements));

orb_elements_dot(5) = n * (1 + e*cos(theta))^2 / (1 - e^2)^(3/2);

== matlab function project/Gyro rafa/Filter/MATLAB Function ==
  data: w_meas input; u input; w_est input; west_dot output
function west_dot = dynamics(w_meas, u, w_est)

% J1 = 0.0547;
% J2 = 0.0519;
% J3 = 0.0574; % https://issfd.org/ISSFD_2014/ISSFD24_Paper_S1-4_carrara.pdf
J1 = 100.9e-2;
J2 =  25.1e-2;
J3 =  91.6e-2;

alpha = 2;

west_dot = zeros(size(w_est));

west_dot(1) = (J2 - J3)/J1*w_est(2)*w_est(3) + u(1)/J1 - ...
                                           alpha*(w_est(1) - w_meas(1))/J1;
west_dot(2) = (J3 - J1)/J2*w_est(1)*w_est(3) + u(2)/J2 - ...
                                           alpha*(w_est(2) - w_meas(2))/J2;
west_dot(3) = (J1 - J2)/J3*w_est(1)*w_est(2) + u(3)/J3 - ...
                                           alpha*(w_est(3) - w_meas(3))/J3;

== matlab function project/Gyro rafa/Gyro model/MATLAB Function ==
  data: x_dot output; x input; w input; M output
function [x_dot, M]= gyro(x, w)

Ir = 1e-7;
Iz = 2e-7;

k = 10;
c = 2*sqrt(k*Iz);

w_x = w(1);
w_y = w(2);
w_z = w(3);
w_r = 100*pi/180;

t_x = x(1); 
t_y = x(2); 
t_z = x(3);
tdot_x = x(4);
tdot_y = x(5); 
tdot_z = x(6); 

x_dot = zeros(6,1);

x_dot(1) = tdot_x;
x_dot(2) = tdot_y; 
x_dot(3) = tdot_z;
x_dot(4) = -(c/Iz)*tdot_x - (k/Iz)*t_x - (Ir/Iz)*w_r*w_x;
x_dot(5) = -(c/Iz)*tdot_y - (k/Iz)*t_y - (Ir/Iz)*w_r*w_y;
x_dot(6) = -(c/Iz)*tdot_z - (k/Iz)*t_z - (Ir/Iz)*w_r*w_z;

M_x = -k*t_x - c*tdot_x;
M_y = -k*t_y - c*tdot_y;
M_z = -k*t_z - c*tdot_z;

M = [M_x M_y M_z]';

== matlab function project/Disturbances: -grav.gradient -airdrag -SRP -magnetic field/gravity gradient/gravity gradient ==
  data: A_BL input; G output; J input; n input
function G = fcn(A_BL,J,n)

%Data
% mu = 3.986004418e14;
% n  = sqrt(mu/a^3);
% %Moment of inertia of s/c
% Ix = 100.9e-2; %[kg m^2]
% Iy = 25.1e-2;
% Iz = 91.6e-2; 
Ix = J(1);
Iy = J(2);
Iz = J(3);
c = A_BL * [1;0;0];

G = zeros(3,1);
G(1) = 3*n^2 * (Iz - Iy)*c(3)*c(2);
G(2) = 3*n^2 * (Ix - Iz)*c(1)*c(3);
G(3) = 3*n^2 * (Iy - Ix)*c(2)*c(1);

end

== matlab function project/Disturbances: -grav.gradient -airdrag -SRP -magnetic field/gravity gradient/A_N//L/MATLAB Function1 ==
  data: t input; A_LN output; n input
function A_LN = fcn(t,n)

% mu = 3.986004418e14;
% n = sqrt( mu / a^3 ); %is this the nº of revolutions per orbit?
A_LN = [cos(n*t) sin(n*t) 0;
    -sin(n*t) cos(n*t) 0;
    0 0 1;
    ];

== matlab function project/RW tracking control/detumblingl control of 1 RW/ideal control to torque of 1 RW ==
  data: u input; h_r_dot output; w input; h_r input; A input
function h_r_dot = fcn(u,w,h_r,A)

Apseudo_inv = pinv(A);

h_r_dot = 0;
h_r_dot = -Apseudo_inv*(u+cross(w,A*h_r));

== matlab function project/reference DCM/DCM_ref ==
  data: v_ref input; A_BN output; r_sc input
function A_BN = DCM_ref (v_ref, r_sc)

r_sc = r_sc/norm(r_sc);

v1 = v_ref/norm(v_ref); 
v3 = cross(v1,r_sc)/norm(cross(v1,r_sc));
v2 = cross(v3,v1);

A_BN = [v2, v3, v1];
